simulink model "admittance_controller_euler"  (R2021b)
settings: Solver=VariableStepAuto  StartTime=0.0  StopTime=10.0  RelTol=1e-3
values from neighbouring files (symbols this model uses):
  ddphi_d = [0 0 0]'    [admittance_controller.m]
  dphi_cd0 = [0 0 0]'    [admittance_controller.m]    (also in sim_admittance_controller.m; simulation_admittance_controller.m)
  dphi_d = [0 0 0]'    [admittance_controller.m]
  Kd = eye(n)*kd    [admittance_controller.m]    (also in sim_admittance_controller.m = eye(3)*kd; sim_invdyn.m = eye(3)*50; simulation_admittance_controller.m = eye(3) * 4; simulation_invdyn.m = eye(3)*50)
  Kp = eye(n)*kp    [admittance_controller.m]    (also in sim_admittance_controller.m = eye(3)*kp; sim_invdyn.m = eye(3)*200; simulation_admittance_controller.m = eye(3) * 16; simulation_invdyn.m = eye(3)*200)
  Md = eye(n)*md    [admittance_controller.m]    (also in sim_admittance_controller.m = eye(3)*md; simulation_admittance_controller.m = eye(3) * 1)
  mu = [1 0.5 1]'    [admittance_controller.m]
  phi_cd0 = [0 0 0]'    [admittance_controller.m]    (also in sim_admittance_controller.m; simulation_admittance_controller.m)
  phi_d = [pi/2 0 pi/4]'    [admittance_controller.m]    (also in sim_admittance_controller.m = rotm2eul(R_ds, "XYZ"))
settings Model: Creator=Martin  LastModifiedBy=Martin

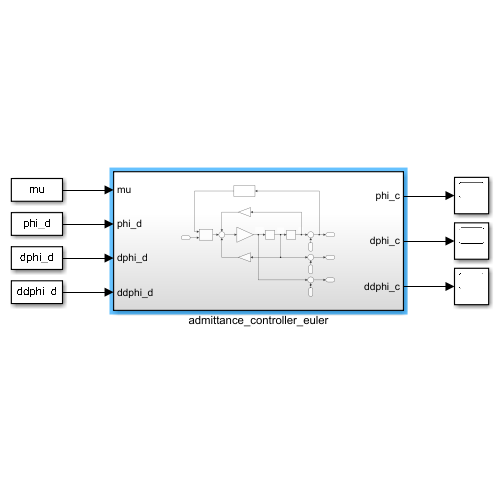
[thumbnail: Simulink's stored preview of the top-level diagram]
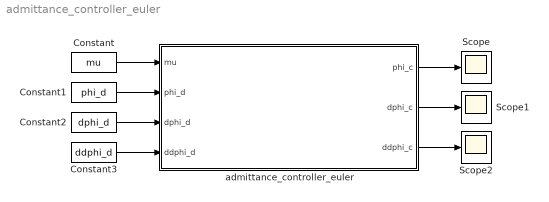
== system admittance_controller_euler ==
  Constant : Constant  Value=mu
  Constant1 : Constant  Value=phi_d
  Constant2 : Constant  Value=dphi_d
  Constant3 : Constant  Value=ddphi_d
  Scope : Scope
  Scope1 : Scope
  Scope2 : Scope
  admittance_controller_euler : Subsystem
  wires:
  Constant/1 -> admittance_controller_euler/1(mu)
  Constant1/1 -> admittance_controller_euler/2(phi_d)
  Constant2/1 -> admittance_controller_euler/3(dphi_d)
  Constant3/1 -> admittance_controller_euler/4(ddphi_d)
  admittance_controller_euler/1(phi_c) -> Scope/1
  admittance_controller_euler/2(dphi_c) -> Scope1/1
  admittance_controller_euler/3(ddphi_c) -> Scope2/1

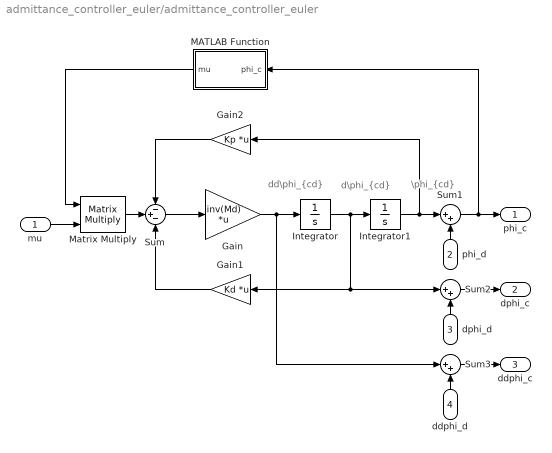
== system admittance_controller_euler/admittance_controller_euler ==
  note: \phi_{cd}
  note: d\phi_{cd}
  note: dd\phi_{cd}
  mu : Inport
  phi_d : Inport  Port=2
  dphi_d : Inport  Port=3
  ddphi_d : Inport  Port=4
  Gain : Gain  Gain=inv(Md)  Multiplication=Matrix(K*u)
  Gain1 : Gain  Gain=Kd  Multiplication=Matrix(K*u)
  Gain2 : Gain  Gain=Kp  Multiplication=Matrix(K*u)
  Integrator : Integrator  InitialCondition=dphi_cd0
  Integrator1 : Integrator  InitialCondition=phi_cd0
  MATLAB Function : MATLAB Function  TreatAsAtomicUnit=on
  Matrix Multiply : Product  Multiplication=Matrix(*)
  Sum : Sum  Inputs=-+-
  Sum1 : Sum  Inputs=|++
  Sum2 : Sum  Inputs=|++
  Sum3 : Sum  Inputs=|++
  phi_c : Outport
  dphi_c : Outport  Port=2
  ddphi_c : Outport  Port=3
  wires:
  Sum2/1 -> dphi_c/1
  Sum3/1 -> ddphi_c/1
  Integrator/1 -> Gain1/1, Sum2/1, Integrator1/1
  Integrator1/1 -> Sum1/1, Gain2/1
  dphi_d/1 -> Sum2/2
  Gain/1 -> Sum3/1, Integrator/1
  ddphi_d/1 -> Sum3/2
  Sum1/1 -> MATLAB Function/1(phi_c), phi_c/1
  phi_d/1 -> Sum1/2
  Sum/1 -> Gain/1
  Gain2/1 -> Sum/1
  Gain1/1 -> Sum/3
  MATLAB Function/1(mu) -> Matrix Multiply/1
  mu/1 -> Matrix Multiply/2
  Matrix Multiply/1 -> Sum/2

== matlab function admittance_controller_euler/MATLAB Function ==
  data: phi_c input; mu output
function mu = T(phi_c)

    phi = phi_c(1); th = phi_c(2); psi = phi_c(3);

    dphi_ = eye(3); dphi_ = dphi_(:, 1);
    dth_  = eye(3) * rotx(phi); dth_ = dth_(:, 2);
    dpsi_ = eye(3) * rotx(phi) * roty(th); dpsi_ = dpsi_(:, 3);
    
    mu = [dphi_ dth_ dpsi_];
    
end
